simulink model "testBusMemory"  (R2014a)
settings: Solver=FixedStepDiscrete  StartTime=0.0  StopTime=Inf  FixedStep=0.001  RelTol=1e-3
libraries: libBusSerialize x1
settings Model: BufferReuse=off  Creator=djoshea  LastModifiedBy=djoshea
settings SolverCC: EnableConcurrentExecution=on
settings OptimizationCC: BlockReduction=off  OptimizeBlockIOStorage=off  BufferReuse=off  GlobalBufferReuse=off  ExpressionFolding=off  LocalBlockOutputs=off
settings HardwareCC: ProdIntDivRoundTo=Zero  ProdEndianess=LittleEndian  ProdHWDeviceType=Generic->32-bit x86 compatible
settings RTWCC: SystemTargetFile=slrt.tlc  TemplateMakefile=slrt_default_tmf  Description=Simulink Real-Time  ProcessScript=slrt_make_rtw_hook  RTWCompilerOptimization=On
settings SimulinkRealTimeCC: GeneratePreprocessorConditionals=Disable all  EnableShiftOperators=on

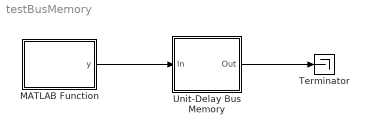
== system testBusMemory ==
  MATLAB Function : MATLAB Function  TreatAsAtomicUnit=on
  Terminator : Terminator
  Unit-Delay Bus Memory : Subsystem  TreatAsAtomicUnit=on  mask(Bus Unit-Delay Memory Block){busType=Bus: RigOutputBus}
      mask prompts: busType "Bus Type:"
      mask help: This block acts exactly like a Memory block and can be used to break algebraic loops. However, unlike Memory blocks, it supports bus signals with variable length bus elements. Internally, this is done by serializing the bus, passing it through a Memory block, and then deserializing at the other end.
      mask init:
      | BusSerialize.maskBusMemoryBlockUpdate(gcb);
      mask Display:
      | text(.5, 0.2, 'Bus Memory', 'HorizontalAlignment', 'center');
      | x = [0.5 0.7 0.7 0.3 0.3 0.25 NaN 0.35 0.3];
      | y = [0.4 0.4 0.8 0.8 0.4 0.45 NaN 0.45 0.4];
      | plot(x, y);
  wires:
  MATLAB Function/1(y) -> Unit-Delay Bus Memory/1(In)
  Unit-Delay Bus Memory/1(Out) -> Terminator/1

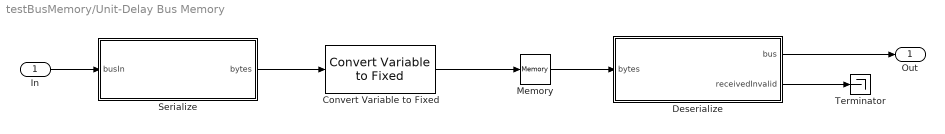
== system testBusMemory/Unit-Delay Bus Memory ==
  In : Inport  OutDataTypeStr=Bus: RigOutputBus  PortDimensions=1
  Convert Variable to Fixed : libBusSerialize/Convert Variable to Fixed  bufferSize=1000
  Deserialize : MATLAB Function  AncestorBlock=libBusSerialize/fn4  TreatAsAtomicUnit=on  mask(BusSerialize: deserialize block){busType=Bus: RigOutputBus}
      mask prompts: busType "Bus Type"
      mask help: Select the bus type below to deserialize into.
      mask init:
      | BusSerialize.maskDeserializeBlockUpdate(gcb)
  Memory : Memory
  Serialize : MATLAB Function  AncestorBlock=libBusSerialize/fn5  TreatAsAtomicUnit=on  mask(BusSerialize: serialize block){busType=Bus: RigOutputBus}
      mask prompts: busType "Bus Type"
      mask help: Select the bus type below to serialize.
      mask init:
      | BusSerialize.maskSerializeBlockUpdate(gcb)
  Terminator : Terminator
  Out : Outport  OutDataTypeStr=Bus: RigOutputBus
  wires:
  Deserialize/1(bus) -> Out/1
  Deserialize/2(receivedInvalid) -> Terminator/1
  In/1 -> Serialize/1(busIn)
  Memory/1 -> Deserialize/1(bytes)
  Serialize/1(bytes) -> Convert Variable to Fixed/1
  Convert Variable to Fixed/1 -> Memory/1

== matlab function testBusMemory/MATLAB Function ==
  data: y output Bus: RigOutputBus size=1
function y = fcn()
%#codegen

y = initializeBus_RigOutputBus();

== matlab function testBusMemory/Unit-Delay Bus Memory/Deserialize ==
  data: bytes input uint8; bus output Bus: RigOutputBus size=1; receivedInvalid output uint8 size=1
function [bus, receivedInvalid] = deserializeWithMemory(bytes)

%#codegen



    % cache input so we only deserialize when input changes

    persistent pBytes;

    if isempty(pBytes)

        pBytes = bytes;

        inChanged = uint8(1);

    elseif ~isequal(pBytes, bytes)

        pBytes = bytes;

        inChanged = uint8(1);

    else

        inChanged = uint8(0);

    end

    

    persistent pInvalid;

    if isempty(pInvalid)

        pInvalid = uint8(0);

    end



    % external cached output

    persistent pBusOut;

    if isempty(pBusOut)

        pBusOut = initializeBus_RigOutputBus();

    end



    % handle deserialization if changed

    if inChanged

        [tempBus, valid] = deserializeBus_RigOutputBus(bytes);

        if valid

            pBusOut = tempBus;

            pInvalid = uint8(0);

        else

            pInvalid = uint8(1);

        end

    end

         

    bus = pBusOut;

    receivedInvalid = pInvalid;

end

== matlab function testBusMemory/Unit-Delay Bus Memory/Serialize ==
  data: busIn input Bus: RigOutputBus size=1; bytes output uint8 size=23125
function bytes = serialize(busIn)
%#codegen, 

    coder.varsize('pBytes', 23125);
    coder.varsize('bytes', 23125);

    persistent pBus;
    persistent pBytes;
    if isempty(pBus)
        pBus = busIn;
        pBytes = zeros(0, 1, 'uint8');
        changed = uint8(1);
        
    elseif ~isequal(pBus, busIn)
        pBus = busIn;
        changed = uint8(1);
    else
        changed = uint8(0);
    end

    if changed
        pBytes = serializeBus_RigOutputBus(busIn);
    end
    
    bytes = pBytes;
end
